simulink subsystem "setArmPositionsInUnreal"  (R2024a)
settings: Solver=VariableStepAuto  StartTime=0.0  StopTime=10.0  RelTol=1e-3
libraries: sim3dlib x4, simulink_extras x4
settings Model: Creator=ckammer  LastModifiedBy=ckammer

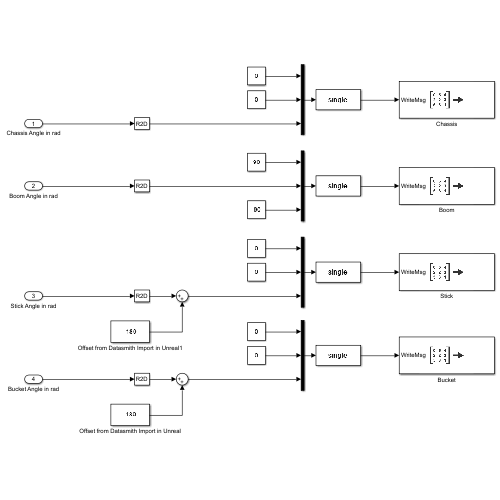
[thumbnail: Simulink's stored preview of the top-level diagram]
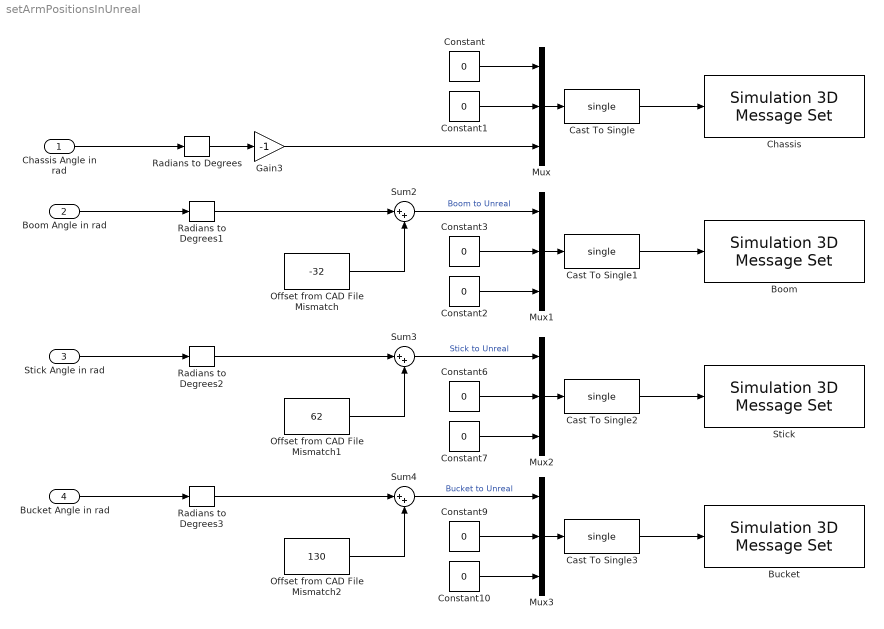
== system setArmPositionsInUnreal ==
  Chassis Angle in rad : Inport
  Boom Angle in rad : Inport  Port=2
  Stick Angle in rad : Inport  Port=3
  Bucket Angle in rad : Inport  Port=4
  Boom : sim3dlib/Simulation 3D Message Set  Priority=-1  SigName=ExcavatorBoomAngle  Ts=-1  aMode=0
      settings: LibrarySourceBlock=aerolibsim3d/Simulation 3D Message Set
  Bucket : sim3dlib/Simulation 3D Message Set  Priority=-1  SigName=ExcavatorBucketAngle  Ts=-1  aMode=0
      settings: LibrarySourceBlock=aerolibsim3d/Simulation 3D Message Set
  Cast To Single{,1..3} (4 alike) : DataTypeConversion  OutDataTypeStr=single  SaturateOnIntegerOverflow=off  RndMeth=Floor
  Chassis : sim3dlib/Simulation 3D Message Set  Priority=-1  SigName=ExcavatorChassisAngle  Ts=-1  aMode=0
      settings: LibrarySourceBlock=aerolibsim3d/Simulation 3D Message Set
  Constant{,1..3,6..7,9..10} (8 alike) : Constant  Value=0  OutDataTypeStr=double
  Gain3 : Gain  Gain=-1
  Mux{,1..3} (4 alike) : Mux  Inputs=3
  Offset from CAD File Mismatch : Constant  Value=-32
  Offset from CAD File Mismatch1 : Constant  Value=62
  Offset from CAD File Mismatch2 : Constant  Value=130
  Radians to Degrees{,1..3} (4 alike) : simulink_extras/Transformations/Radians to Degrees
  Stick : sim3dlib/Simulation 3D Message Set  Priority=-1  SigName=ExcavatorStickAngle  Ts=-1  aMode=0
      settings: LibrarySourceBlock=aerolibsim3d/Simulation 3D Message Set
  Sum2 : Sum  Inputs=|++
  Sum3 : Sum  Inputs=|++
  Sum4 : Sum  Inputs=|++
  wires:
  Mux2/1 -> Cast To Single2/1
  Radians to Degrees/1 -> Gain3/1
  Mux3/1 -> Cast To Single3/1
  Mux1/1 -> Cast To Single1/1
  Cast To Single3/1 -> Bucket/1
  Cast To Single1/1 -> Boom/1
  Constant1/1 -> Mux/2
  Cast To Single2/1 -> Stick/1
  Mux/1 -> Cast To Single/1
  Cast To Single/1 -> Chassis/1
  Constant/1 -> Mux/1
  Chassis Angle in rad/1 -> Radians to Degrees/1
  Boom Angle in rad/1 -> Radians to Degrees1/1
  Stick Angle in rad/1 -> Radians to Degrees2/1
  Bucket Angle in rad/1 -> Radians to Degrees3/1
  Offset from CAD File Mismatch/1 -> Sum2/2
  Offset from CAD File Mismatch1/1 -> Sum3/2
  Offset from CAD File Mismatch2/1 -> Sum4/2
  Sum2/1 -> Mux1/1  "Boom to Unreal"
  Constant3/1 -> Mux1/2
  Constant2/1 -> Mux1/3
  Sum3/1 -> Mux2/1  "Stick to Unreal"
  Constant6/1 -> Mux2/2
  Constant7/1 -> Mux2/3
  Sum4/1 -> Mux3/1  "Bucket to Unreal"
  Constant9/1 -> Mux3/2
  Constant10/1 -> Mux3/3
  Radians to Degrees2/1 -> Sum3/1
  Radians to Degrees3/1 -> Sum4/1
  Radians to Degrees1/1 -> Sum2/1
  Gain3/1 -> Mux/3
